simulink model "Test_SG_circuit_exc_turb"  (R2020b)
settings: Solver=ode1  StartTime=0.0  StopTime=15  FixedStep=10e-6  RelTol=1e-3
values from neighbouring files (symbols this model uses):
  L1d_pu = Lb/Lbase    [SG_param.m]    (also in SG_param_tool.m; SG_param_tool_POD.m = (Xd_subtr-Xl)*(Lmd_pu*Lfd_pu)/(Lmd_pu*Lfd_pu-(Lfd_pu+Lmd_pu))
  L1q_pu = La/Lbase    [SG_param.m]    (also in SG_param_tool.m; SG_param_tool_POD.m = (Lmq_pu*(Xq_tr-Xl))/(Lmq_pu-Xq_tr+Xl))
  L2q_pu = Lb/Lbase    [SG_param.m]    (also in SG_param_tool.m; SG_param_tool_POD.m = (Xq_subtr-Xl)*(Lmq_pu*L1q_pu)/(Lmq_pu*L1q_pu-(L1q_pu+Lmq_pu))
  Lfd_pu = La/Lbase    [SG_param.m]    (also in SG_param_tool.m; SG_param_tool_POD.m = (Lmd_pu*(Xd_tr-Xl))/(Lmd_pu-Xd_tr+Xl))
  Ll_pu = Xl    (= 0.2)    [SG_param.m]    (also in SG_param_tool.m; SG_param_tool_POD.m = Xl)
  Lmd_pu = Xd - Xl    (= 1.6)    [SG_param.m]    (also in SG_param_tool.m; SG_param_tool_POD.m = Xd - Xl)
  Lmq_pu = Xq - Xl    (= 1.5)    [SG_param.m]    (also in SG_param_tool.m; SG_param_tool_POD.m = Xq - Xl)
  Pm = Psg0+(Iq.^2+Id.^2)*Rs_pu    [Init_values_Simulink.m]    (also in Init_values_Simulink_trafo.m)
  R1d_pu = rb/Zb    [SG_param.m]    (also in SG_param_tool.m; SG_param_tool_POD.m = 1/(Tdo_subtr*wb)*(L1d_pu+Lmd_pu*Lfd_pu/(Lmd_pu+Lfd_pu)))
  R1q_pu = ra/Zb    [SG_param.m]    (also in SG_param_tool.m; SG_param_tool_POD.m = (Lmq_pu+L1q_pu)/(Tqo_tr*wb))
  R2q_pu = rb/Zb    [SG_param.m]    (also in SG_param_tool.m; SG_param_tool_POD.m = 1/(Tqo_subtr*wb)*(L2q_pu+Lmq_pu*L1q_pu/(Lmq_pu+L1q_pu)))
  Rf_pu = ra/Zb    [SG_param.m]    (also in SG_param_tool.m; SG_param_tool_POD.m = (Lmd_pu+Lfd_pu)/(Tdo_tr*wb))
  Rs_pu = 0.0025    [SG_param.m]    (also in SG_param_tool.m; SG_param_tool_POD.m)
  Rsnb = 300    [SG_param.m]    (also in SG_param_tool.m; SG_param_tool_POD.m; SS_model_grid.m = Vn^2/(data.SG(ii,2)*1e6*0.01)*Ssnb(ii))
  Vb = 22e3    (= 22000)    [SG_param.m]    (also in sg_slack_POD.m = Vb_kV*1e3)
  Vf = Efd    [Init_values_Simulink.m]    (also in Init_values_Simulink_trafo.m)
  Vref = Efd/Exc.KA+V    [Init_values_Simulink.m]    (also in Init_values_Simulink_trafo.m = Vf/Exc.KA+V; Initial_values_for_linear_model.m = Efd/Exc.KA+abs(Vin))
  wn = 2*pi*fn    (= 314.159265359)    [SG_param.m]
undefined symbols (not defined in the file or in its folder): Exc, Lg, Rg, tstep
libraries: powerlib x41, simulink_extras x9, powerlib_meascontrol x2
(part 2 of 2)

== system Test_SG_circuit_exc_turb/Exciter System/SEXS1 ==
  note: The controller parameters provided by ENTSO-E
      | define different names for the parameters:
      |
      | ENTSO-E = IEEE Std 421.5-2005
      | Ta = Tc
      | Tb = Tb
      | K = Ka
      | Te = Ta
      | Emax = Vrmax
      | Emin = Vrmin
  note: The exciter model provided by ENTSO-E most similar to the IEEE is the Type AC4A excitation system model
  Vref : Inport
  Vc : Inport  Port=2
  Vs : Inport  Port=3
  Saturation : Saturate  UpperLimit=Emax  LowerLimit=Emin
  Sum : Sum  Inputs=+-+
  Transfer Fcn (with initial outputs) : simulink_extras/Additional Linear/Transfer Fcn (with initial outputs)  N=[K]  D=[Te 1]  Y0=Vf0  U0=Vf0/K
  Transfer Fcn (with initial outputs)1 : simulink_extras/Additional Linear/Transfer Fcn (with initial outputs)  N=[Ta 1]  D=[Tb 1]  Y0=Vf0/K  U0=Vf0/K
  Efd : Outport
  wires:
  Saturation/1 -> Efd/1  "vfd"
  Transfer Fcn (with initial outputs)/1 -> Saturation/1
  Transfer Fcn (with initial outputs)1/1 -> Transfer Fcn (with initial outputs)/1
  Sum/1 -> Transfer Fcn (with initial outputs)1/1
  Vs/1 -> Sum/3
  Vref/1 -> Sum/1
  Vc/1 -> Sum/2

== system Test_SG_circuit_exc_turb/Exciter System/TR and LC_test ==
  note: Rc and Xc should be negative values in case of voltage regulated after an impedance
  note: Fig 4.1 of IEEE Std 421.5-2005
  note: Vt and It should be phasors (complex quantities)
  note: compensated
      | impedance
  note: Terminal voltage transducer and optional load compensation
  Vt : Inport
  It : Inport  Port=2
  Abs : Abs
  Abs1 : Abs
  Rc+jXc : Gain  Gain=abs(Rc+1i*Xc)
  Saturation : Saturate  UpperLimit=12  LowerLimit=-100.8
  Scope : Scope
  Sum : Sum  Inputs=|+-
  Transfer Fcn (with initial outputs) : simulink_extras/Additional Linear/Transfer Fcn (with initial outputs)  N=[1]  D=[Tr 1]  Y0=1  U0=1
  Vc : Outport
  wires:
  Abs1/1 -> Rc+jXc/1
  Abs/1 -> Sum/1
  It/1 -> Abs1/1
  Sum/1 -> Transfer Fcn (with initial outputs)/1
  Rc+jXc/1 -> Sum/2
  Transfer Fcn (with initial outputs)/1 -> Scope/1, Saturation/1
  Vt/1 -> Abs/1
  Saturation/1 -> Vc/1
